simulink model "q_rotpen_mdl_student"  (Simulink 9.1)
settings: Solver=ode1  StartTime=0.0  StopTime=inf  FixedStep=0.002  RelTol=1e-3  EnableMultiTasking=on
PostLoadFcn:
  | qc_set_target_type(getConfigSet(bdroot, 'QUARC Default Target Configuration'));
values from neighbouring files (symbols this model uses):
  K_AMP = 1    [setup_rotpen.m]
undefined symbols (not defined in the file or in its folder): HIL, K_ENC
libraries: quarc_library x5, simulink_extras x2
settings Model: Creator=MLevis  LastModifiedBy=hopeg1  SimulationMode=external  ExtModeTrigDuration=10000
settings SolverCC: PositivePriorityOrder=on
settings DataIOCC: LimitDataPoints=on  SignalLoggingSaveFormat=ModelDataLogs
settings OptimizationCC: ExpressionDepthLimit=2147483647  InitFltsAndDblsToZero=on
settings DebuggingCC: SaveWithParameterizedLinksMsg=none  SolverPrmCheckMsg=warning  MultiTaskDSMMsg=warning  MultiTaskCondExecSysMsg=none  FcnCallInpInsideContextMsg=warning  StateNameClashWarn=warning
settings RTWCC: SystemTargetFile=quarc_win64.tlc  TemplateMakefile=quarc_default_tmf  Description=QUARC Win64 Target
settings STFCustomTargetCC: TargetPreCompLibLocation=C:\PROGRA~3\QUARC\lib\2011a\win64\release  ConcurrentExecutionCompliant=on  GeneratePreprocessorConditionals=Disable all  CPPClassGenCompliant=on  SystemTargetFile=quarc_win64.tlc
settings GRTTargetCC: TargetPreCompLibLocation=C:\PROGRA~3\QUARC\lib\2018a\win64\release  ParMdlRefBuildCompliant=off  CompOptLevelCompliant=off  GeneratePreprocessorConditionals=Disable all  MatFileLogging=off  UseToolchainInfoCompliant=off  ExtMode=on  ExtModeMexFile=quarc_comm

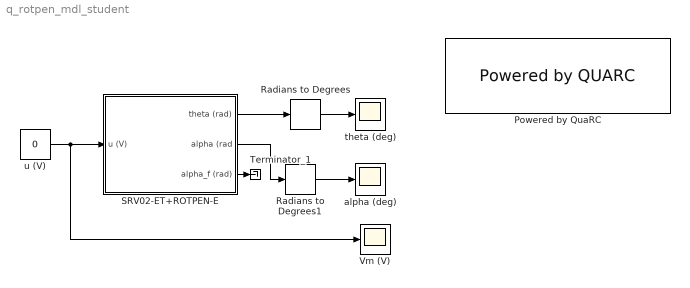
== system q_rotpen_mdl_student ==
  Powered by QuaRC : quarc_library/Logos/Powered by QUARC
  Radians to Degrees : simulink_extras/Transformations/Radians to Degrees
  Radians to Degrees1 : simulink_extras/Transformations/Radians to Degrees
  SRV02-ET+ROTPEN-E : Subsystem
  Terminator_1 : Terminator
  Vm (V) : Scope
  alpha (deg) : Scope
  theta (deg) : Scope
  u (V) : Constant  Value=0
  wires:
  u (V)/1 -> SRV02-ET+ROTPEN-E/1(u (V)), Vm (V)/1
  SRV02-ET+ROTPEN-E/3(alpha_f (rad)) -> Terminator_1/1
  SRV02-ET+ROTPEN-E/1(theta (rad)) -> Radians to Degrees/1
  SRV02-ET+ROTPEN-E/2(alpha (rad) -> Radians to Degrees1/1
  Radians to Degrees/1 -> theta (deg)/1
  Radians to Degrees1/1 -> alpha (deg)/1

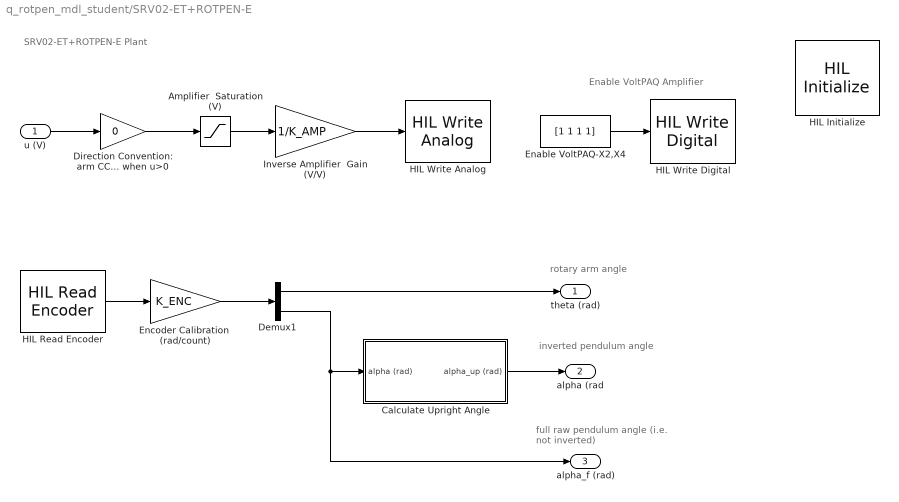
== system q_rotpen_mdl_student/SRV02-ET+ROTPEN-E ==
  note: SRV02-ET+ROTPEN-E Plant
  note: Enable VoltPAQ Amplifier
  note: inverted pendulum angle
  note: rotary arm angle
  note: full raw pendulum angle
      |  (i.e. not inverted)
  u (V) : Inport
  Amplifier  Saturation (V) : Saturate  UpperLimit=5  LowerLimit=-5
  Calculate Upright Angle : Subsystem
  Demux1 : Demux  Outputs=2
  Direction Convention: arm CCW when u>0 : Gain  Gain=0  SaturateOnIntegerOverflow=on  OutDataTypeStr=Inherit: Same as input  ParamDataTypeStr=Inherit: Same as input
  Enable VoltPAQ-X2,X4 : Constant  Value=[1 1 1 1]
  Encoder Calibration  (rad/count) : Gain  Gain=K_ENC  SaturateOnIntegerOverflow=on  OutDataTypeStr=Inherit: Same as input  ParamDataTypeStr=Inherit: Same as input
  HIL Initialize : quarc_library/Data Acquisition/Generic/Configuration/HIL Initialize  object_name=HIL-1  board_type=q8_usb  board_number=0  board_options=update_rate=normal  exclusive=off  active=off  hardware_clocks=[0:2]  clock_modes=[]  initial_clock_frequencies=[]  set_clock_params_at_start=off  set_clock_params_at_switch_in=off  set_clock_frequencies_at_start=off  set_clock_frequencies_at_switch_in=off  analog_input_channels=[0:7]  analog_input_configurations=[]  analog_input_maximums=10  analog_input_minimums=-10  set_analog_input_params_at_start=on  set_analog_input_params_at_switch_in=off  analog_output_channels=[0]  analog_output_maximums=10  analog_output_minimums=-10  initial_analog_outputs=[0]  final_analog_outputs=[0]  watchdog_analog_outputs=0  set_analog_output_params_at_start=on  set_analog_output_params_at_switch_in=off  set_analog_outputs_at_start=on  set_analog_outputs_at_switch_in=off  set_analog_outputs_at_terminate=on  set_analog_outputs_at_switch_out=off  set_analog_outputs_on_watchdog=off  digital_input_channels=[]  digital_output_channels=[1]  digital_output_configuration=[]  initial_digital_outputs=[1]  final_digital_outputs=[0]  watchdog_digital_outputs=[0]  set_digital_output_params_at_start=off  set_digital_output_params_at_switch_in=off  set_digital_outputs_at_start=on  set_digital_outputs_at_switch_in=off  set_digital_outputs_at_terminate=on  set_digital_outputs_at_switch_out=off  set_digital_outputs_on_watchdog=off  encoder_channels=[0:1]  quadrature=[4]  encoder_filter_frequency=[]  initial_encoder_counts=[0]  set_encoder_params_at_start=on  set_encoder_params_at_switch_in=off  set_encoder_counts_at_start=on  set_encoder_counts_at_switch_in=off  pwm_channels=[0:1]  pwm_modes=0  pwm_frequency=99.532799999999995e6/4095  pwm_configuration=[0]  pwm_alignment=[0]  pwm_polarity=[1]  pwm_leading_deadband=[0]  pwm_trailing_deadband=[0]  initial_pwm_outputs=[0]  final_pwm_outputs=[0]  watchdog_pwm_outputs=[0]  set_pwm_params_at_start=on  set_pwm_params_at_switch_in=off  set_pwm_outputs_at_start=on  set_pwm_outputs_at_switch_in=off  set_pwm_outputs_at_terminate=on  set_pwm_outputs_at_switch_out=off  set_pwm_outputs_on_watchdog=off  other_output_channels=[]  initial_other_outputs=[]  final_other_outputs=[]  watchdog_other_outputs=[]  set_other_outputs_at_start=off  set_other_outputs_at_switch_in=off  set_other_outputs_at_terminate=off  set_other_outputs_at_switch_out=off  set_other_outputs_on_watchdog=off
  HIL Read Encoder : quarc_library/Data Acquisition/Generic/Immediate I//O/HIL Read Encoder  object_name=HIL-1  channels=[0:1]  sample_time=qc_get_step_size  active=on  vector_output=on  data_type_mode=Inherit via back propagation  data_type=double
  HIL Write Analog : quarc_library/Data Acquisition/Generic/Immediate I//O/HIL Write Analog  object_name=HIL-1  channels=0  sample_time=-1  active=off  vector_input=off
  HIL Write Digital : quarc_library/Data Acquisition/Generic/Immediate I//O/HIL Write Digital  object_name=HIL-1  channels=[0:3]  sample_time=-1  active=off  vector_input=on
      settings: SourceProductName=QUARC Targets
  Inverse Amplifier  Gain (V/V) : Gain  Gain=1/K_AMP
  theta (rad) : Outport
  alpha (rad : Outport  Port=2
  alpha_f (rad) : Outport  Port=3
  wires:
  Encoder Calibration  (rad/count)/1 -> Demux1/1
  Demux1/2 -> Calculate Upright Angle/1(alpha (rad)), alpha_f (rad)/1
  Enable VoltPAQ-X2,X4/1 -> HIL Write Digital/1
  HIL Read Encoder/1 -> Encoder Calibration  (rad/count)/1
  Amplifier  Saturation (V)/1 -> Inverse Amplifier  Gain (V/V)/1
  Inverse Amplifier  Gain (V/V)/1 -> HIL Write Analog/1
  u (V)/1 -> Direction Convention: arm CCW when u>0/1
  Direction Convention: arm CCW when u>0/1 -> Amplifier  Saturation (V)/1
  Demux1/1 -> theta (rad)/1
  Calculate Upright Angle/1(alpha_up (rad)) -> alpha (rad/1

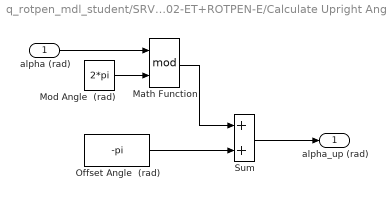
== system q_rotpen_mdl_student/SRV02-ET+ROTPEN-E/Calculate Upright Angle ==
  alpha (rad) : Inport
  Math Function : Math  Operator=mod  SaturateOnIntegerOverflow=on
  Mod Angle  (rad) : Constant  Value=2*pi
  Offset Angle  (rad) : Constant  Value=-pi
  Sum : Sum  SaturateOnIntegerOverflow=on  InputSameDT=on  OutDataTypeStr=Inherit: Same as first input
  alpha_up (rad) : Outport
  wires:
  Sum/1 -> alpha_up (rad)/1
  Mod Angle  (rad)/1 -> Math Function/2
  Offset Angle  (rad)/1 -> Sum/2
  alpha (rad)/1 -> Math Function/1
  Math Function/1 -> Sum/1
